simulink model "TrafficLightDecisionLogic"  (R2022b)
settings: Solver=ode23tb  StartTime=0.0  StopTime=scenario.StopTime  FixedStep=0.001  RelTol=1e-8  EnableMultiTasking=on
undefined symbols (not defined in the file or in its folder): maxMIOLeadDistance, posSelector, referencePathSwitchThreshold, Ts, velSelector
settings Model: Creator=The MathWorks, Inc.  LastModifiedBy=The MathWorks, Inc.
settings SolverCC: ZeroCrossAlgorithm=Adaptive  AlgebraicLoopSolver=TrustRegion  PositivePriorityOrder=on  AutoInsertRateTranBlk=on  InsertRTBMode=Always  DecoupledContinuousIntegration=on  MinimalZcImpactIntegration=on  MaxZcPerStep=1
settings DataIOCC: SaveOutput=off  SaveTime=off  ReturnWorkspaceOutputs=off
settings DebuggingCC: ParameterPrecisionLossMsg=none  UnconnectedInputMsg=warning  UnconnectedOutputMsg=warning  UnconnectedLineMsg=warning  PregeneratedLibrarySubsystemCodeDiagnostic=none  SFMachineParentedDataDiag=warning  ArithmeticOperatorsInVariantConditions=warning
settings HardwareCC: ProdLongLongMode=on
settings ModelReferenceCC: EnableRefExpFcnMdlSchedulingChecks=on
settings SFSimCC: SimUseLocalCustomCode=off
settings RTWCC: GenerateReport=on  RTWUseLocalCustomCode=off  LaunchReport=on  DLArmComputeVersion=19.05
settings ConfigComp: CovScope=ReferencedModels  CovIncludeTopModel=off

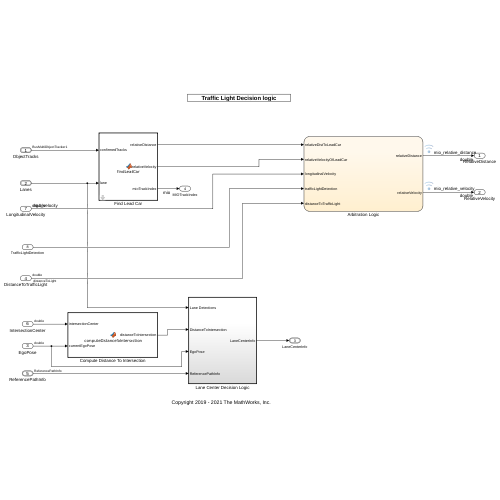
[thumbnail: Simulink's stored preview of the top-level diagram]
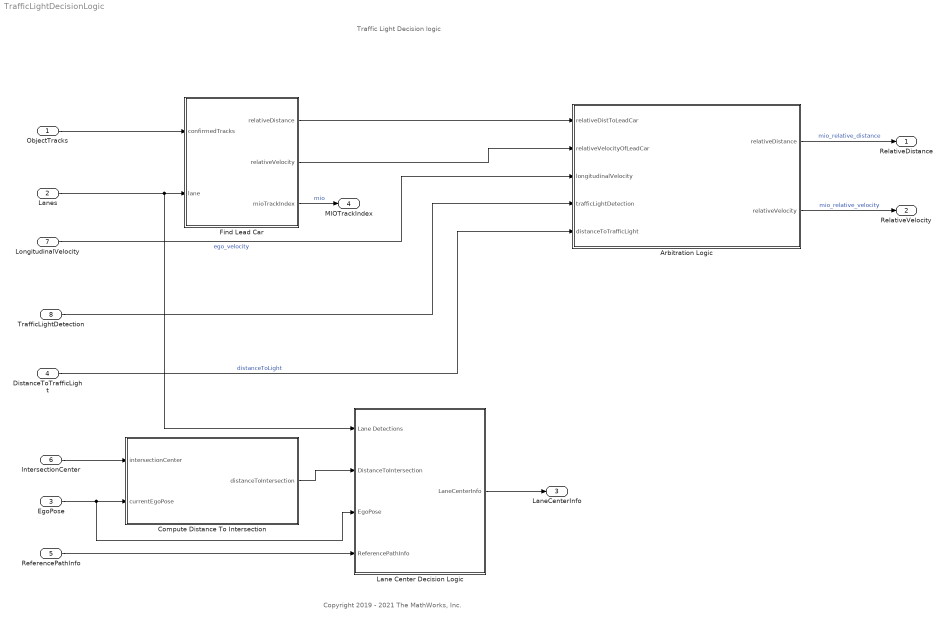
== system TrafficLightDecisionLogic ==
  note: Traffic Light Decision logic
  note: Copyright 2019 - 2021 The MathWorks, Inc.
  ObjectTracks : Inport  OutDataTypeStr=Bus: BusMultiObjectTracker1  PortDimensions=[1 1]  SampleTime=[0.10000000000000001,0]  BusOutputAsStruct=on
  Lanes : Inport  Port=2  OutDataTypeStr=Bus: LaneSensor
  "EgoPose " : Inport  Port=3  OutDataTypeStr=double  PortDimensions=3  SampleTime=[0.10000000000000001,0]
  DistanceToTrafficLight : Inport  Port=4  OutDataTypeStr=double  PortDimensions=1  SampleTime=[0.10000000000000001,0]
  "ReferencePathInfo " : Inport  Port=5  OutDataTypeStr=Bus: ReferencePathInfo  PortDimensions=1  SampleTime=[0.10000000000000001,0]  BusOutputAsStruct=on
  IntersectionCenter : Inport  Port=6  OutDataTypeStr=double  PortDimensions=3  SampleTime=[0.10000000000000001,0]
  LongitudinalVelocity : Inport  Port=7  OutDataTypeStr=double  PortDimensions=1  SampleTime=[0.10000000000000001,0]
  TrafficLightDetection : Inport  Port=8
  Arbitration Logic : Stateflow chart  TreatAsAtomicUnit=on  SystemSampleTime=Ts
  Compute Distance To Intersection : MATLAB Function  TreatAsAtomicUnit=on
  Find Lead Car : MATLAB Function  TreatAsAtomicUnit=on  SystemSampleTime=Ts  mask{positionSelector=posSelector, velocitySelector=velSelector, maxDistance=maxMIOLeadDistance}
      mask prompts: positionSelector "Track position selector"; velocitySelector "Track velocity selector"; maxDistance "Maximum lead distance"
  Lane Center Decision Logic : Subsystem  TreatAsAtomicUnit=on  VariantControl=v2
      settings: RTWFileNameOpts=Use function name
  RelativeDistance : Outport  OutDataTypeStr=double  PortDimensions=1  SampleTime=[0.10000000000000001,0]  VectorParamsAs1DForOutWhenUnconnected=off
  RelativeVelocity : Outport  Port=2  OutDataTypeStr=double  PortDimensions=1  SampleTime=[0.10000000000000001,0]  VectorParamsAs1DForOutWhenUnconnected=off
  LaneCenterInfo : Outport  Port=3  OutDataTypeStr=Bus: BusLaneCenter
  MIOTrackIndex : Outport  Port=4
  wires:
  IntersectionCenter/1 -> Compute Distance To Intersection/1(intersectionCenter)
  LongitudinalVelocity/1 -> Arbitration Logic/3(longitudinalVelocity)  "ego_velocity"
  "ReferencePathInfo "/1 -> Lane Center Decision Logic/4(ReferencePathInfo)
  ObjectTracks/1 -> Find Lead Car/1(confirmedTracks)
  Lanes/1 -> Lane Center Decision Logic/1(Lane Detections), Find Lead Car/2(lane)
  Find Lead Car/3(mioTrackIndex) -> MIOTrackIndex/1  "mio"
  "EgoPose "/1 -> Lane Center Decision Logic/3(EgoPose), Compute Distance To Intersection/2(currentEgoPose)
  Arbitration Logic/1(relativeDistance) -> RelativeDistance/1  "mio_relative_distance"
  Arbitration Logic/2(relativeVelocity) -> RelativeVelocity/1  "mio_relative_velocity"
  Compute Distance To Intersection/1(distanceToIntersection) -> Lane Center Decision Logic/2(DistanceToIntersection)
  Lane Center Decision Logic/1(LaneCenterInfo) -> LaneCenterInfo/1
  TrafficLightDetection/1 -> Arbitration Logic/4(trafficLightDetection)
  Find Lead Car/2(relativeVelocity) -> Arbitration Logic/2(relativeVelocityOfLeadCar)
  DistanceToTrafficLight/1 -> Arbitration Logic/5(distanceToTrafficLight)  "distanceToLight"
  Find Lead Car/1(relativeDistance) -> Arbitration Logic/1(relativeDistToLeadCar)

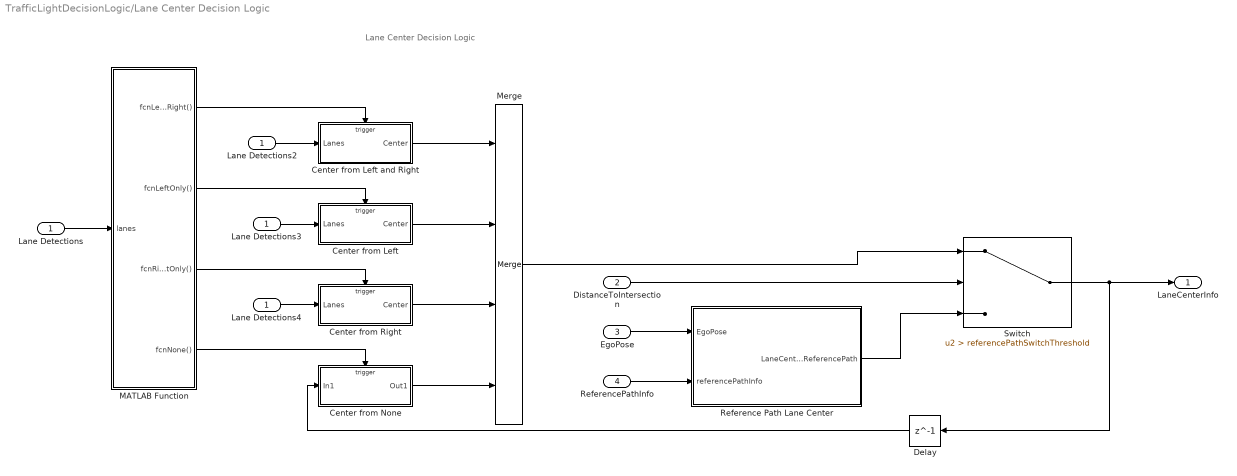
== system TrafficLightDecisionLogic/Lane Center Decision Logic ==
  note: Lane Center Decision Logic
  Lane Detections : Inport
  DistanceToIntersection : Inport  Port=2
  EgoPose : Inport  Port=3
  ReferencePathInfo : Inport  Port=4
  Center from Left : Subsystem  TreatAsAtomicUnit=on
  Center from Left and Right : Subsystem  TreatAsAtomicUnit=on
  Center from None : Subsystem  TreatAsAtomicUnit=on
  Center from Right : Subsystem  TreatAsAtomicUnit=on
  Delay : Delay  DelayLength=1
  Lane Detections2 : InportShadow
  Lane Detections3 : InportShadow
  Lane Detections4 : InportShadow
  MATLAB Function : MATLAB Function  TreatAsAtomicUnit=on
  Merge : Merge  Inputs=4
  Reference Path Lane Center : Subsystem
  Switch : Switch  Criteria=u2 > Threshold  Threshold=referencePathSwitchThreshold  SaturateOnIntegerOverflow=off  InputSameDT=off
      settings: AttributesFormatString=|
      | ----------------------------------------
      | Threshold = %<Threshold>
  LaneCenterInfo : Outport  VectorParamsAs1DForOutWhenUnconnected=off
  wires:
  Center from Right/1(Center) -> Merge/3
  Lane Detections3/1 -> Center from Left/1(Lanes)
  Lane Detections4/1 -> Center from Right/1(Lanes)
  MATLAB Function/2(fcnLeftOnly()) -> Center from Left/Trigger
  MATLAB Function/1(fcnLeftAndRight()) -> Center from Left and Right/Trigger
  Delay/1 -> Center from None/1(In1)
  Center from Left and Right/1(Center) -> Merge/1
  Lane Detections/1 -> MATLAB Function/1(lanes)
  Lane Detections2/1 -> Center from Left and Right/1(Lanes)
  MATLAB Function/3(fcnRightOnly()) -> Center from Right/Trigger
  MATLAB Function/4(fcnNone()) -> Center from None/Trigger
  Center from Left/1(Center) -> Merge/2
  Center from None/1(Out1) -> Merge/4
  ReferencePathInfo/1 -> Reference Path Lane Center/2(referencePathInfo)
  Reference Path Lane Center/1(LaneCenterFromReferencePath) -> Switch/3
  Merge/1 -> Switch/1
  Switch/1 -> LaneCenterInfo/1, Delay/1
  EgoPose/1 -> Reference Path Lane Center/1("EgoPose ")
  DistanceToIntersection/1 -> Switch/2

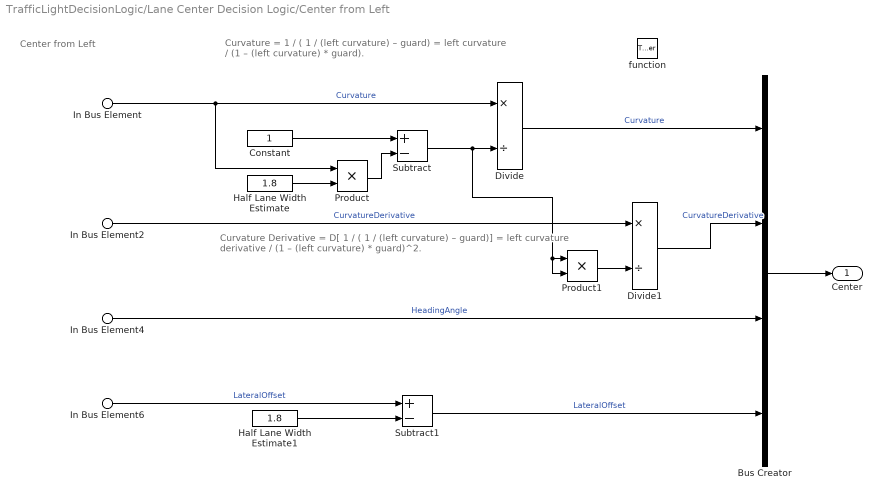
== system TrafficLightDecisionLogic/Lane Center Decision Logic/Center from Left ==
  note: Curvature Derivative
      | = D[ 1 / ( 1 / (left curvature) – guard)]
      | = left curvature derivative / (1 – (left curvature) * guard)^2.
  note: Center from Left
  note: Curvature
      | = 1 / ( 1 / (left curvature) – guard)
      | = left curvature / (1 – (left curvature) * guard).
  In Bus Element : Inport  PortName=Lanes  Element=Left.Curvature
  In Bus Element2 : Inport  PortName=Lanes  Element=Left.CurvatureDerivative
  In Bus Element4 : Inport  PortName=Lanes  Element=Left.HeadingAngle
  In Bus Element6 : Inport  PortName=Lanes  Element=Left.LateralOffset
  function : TriggerPort  TriggerType=function-call  VariantControl=Variant
  Bus Creator : BusCreator  Inputs=4
  Constant : Constant  OutDataTypeStr=Inherit: Inherit via back propagation
  Divide : Product  Inputs=*/
  Divide1 : Product  Inputs=*/
  Half Lane Width Estimate : Constant  Value=1.8  OutDataTypeStr=Inherit: Inherit via back propagation
  Half Lane Width Estimate1 : Constant  Value=1.8  OutDataTypeStr=Inherit: Inherit via back propagation
  Product : Product
  Product1 : Product
  Subtract : Sum  Inputs=+-
  Subtract1 : Sum  Inputs=+-
  Center : Outport  VectorParamsAs1DForOutWhenUnconnected=off
  wires:
  Product/1 -> Subtract/2
  Half Lane Width Estimate1/1 -> Subtract1/2
  In Bus Element6/1 -> Subtract1/1  "LateralOffset"
  Product1/1 -> Divide1/2
  In Bus Element2/1 -> Divide1/1  "CurvatureDerivative"
  Constant/1 -> Subtract/1
  Half Lane Width Estimate/1 -> Product/2
  Subtract/1 -> Divide/2, Product1/1, Product1/2
  In Bus Element/1 -> Divide/1, Product/1  "Curvature"
  Subtract1/1 -> Bus Creator/4  "LateralOffset"
  In Bus Element4/1 -> Bus Creator/3  "HeadingAngle"
  Divide/1 -> Bus Creator/1  "Curvature"
  Divide1/1 -> Bus Creator/2  "CurvatureDerivative"
  Bus Creator/1 -> Center/1

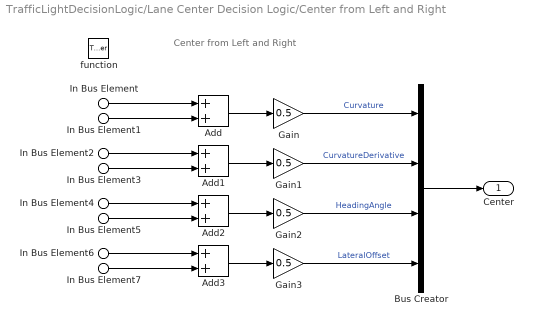
== system TrafficLightDecisionLogic/Lane Center Decision Logic/Center from Left and Right ==
  note: Center from Left and Right
  In Bus Element : Inport  PortName=Lanes  Element=Left.Curvature
  In Bus Element2 : Inport  PortName=Lanes  Element=Left.CurvatureDerivative
  In Bus Element4 : Inport  PortName=Lanes  Element=Left.HeadingAngle
  In Bus Element6 : Inport  PortName=Lanes  Element=Left.LateralOffset
  In Bus Element1 : Inport  PortName=Lanes  Element=Right.Curvature
  In Bus Element3 : Inport  PortName=Lanes  Element=Right.CurvatureDerivative
  In Bus Element5 : Inport  PortName=Lanes  Element=Right.HeadingAngle
  In Bus Element7 : Inport  PortName=Lanes  Element=Right.LateralOffset
  function : TriggerPort  TriggerType=function-call  VariantControl=Variant
  Add{,1..3} (4 alike) : Sum
  Bus Creator : BusCreator  Inputs=4
  Gain{,1..3} (4 alike) : Gain  Gain=0.5
  Center : Outport  VectorParamsAs1DForOutWhenUnconnected=off
  wires:
  In Bus Element6/1 -> Add3/1
  In Bus Element7/1 -> Add3/2
  In Bus Element5/1 -> Add2/2
  In Bus Element4/1 -> Add2/1
  In Bus Element3/1 -> Add1/2
  In Bus Element2/1 -> Add1/1
  In Bus Element1/1 -> Add/2
  In Bus Element/1 -> Add/1
  Bus Creator/1 -> Center/1
  Gain3/1 -> Bus Creator/4  "LateralOffset"
  Add3/1 -> Gain3/1
  Gain2/1 -> Bus Creator/3  "HeadingAngle"
  Add2/1 -> Gain2/1
  Gain1/1 -> Bus Creator/2  "CurvatureDerivative"
  Add1/1 -> Gain1/1
  Gain/1 -> Bus Creator/1  "Curvature"
  Add/1 -> Gain/1

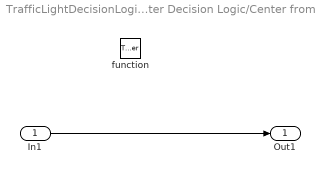
== system TrafficLightDecisionLogic/Lane Center Decision Logic/Center from None ==
  In1 : Inport
  function : TriggerPort  TriggerType=function-call  VariantControl=Variant
  Out1 : Outport  VectorParamsAs1DForOutWhenUnconnected=off
  wires:
  In1/1 -> Out1/1

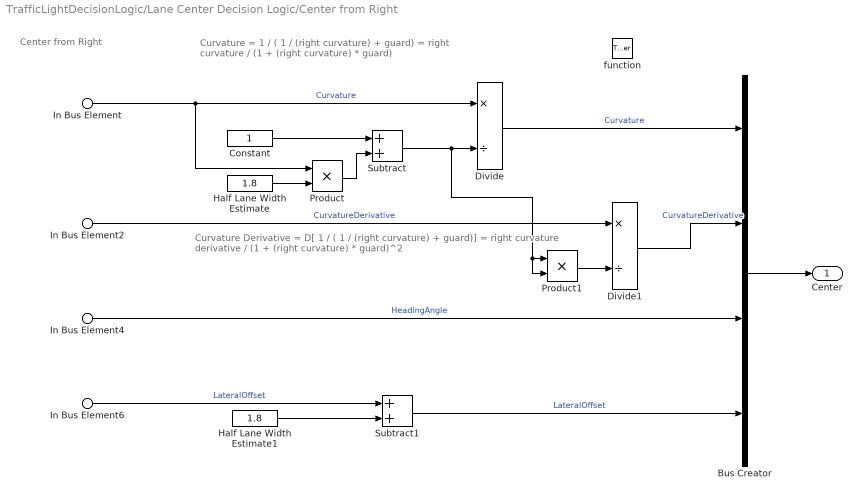
== system TrafficLightDecisionLogic/Lane Center Decision Logic/Center from Right ==
  note: Curvature Derivative
      | = D[ 1 / ( 1 / (right curvature) + guard)]
      | = right curvature derivative / (1 + (right curvature) * guard)^2
  note: Curvature
      | = 1 / ( 1 / (right curvature) + guard)
      | = right curvature / (1 + (right curvature) * guard)
  note: Center from Right
  In Bus Element : Inport  PortName=Lanes  Element=Right.Curvature
  In Bus Element2 : Inport  PortName=Lanes  Element=Right.CurvatureDerivative
  In Bus Element4 : Inport  PortName=Lanes  Element=Right.HeadingAngle
  In Bus Element6 : Inport  PortName=Lanes  Element=Right.LateralOffset
  function : TriggerPort  TriggerType=function-call  VariantControl=Variant
  Bus Creator : BusCreator  Inputs=4
  Constant : Constant  OutDataTypeStr=Inherit: Inherit via back propagation
  Divide : Product  Inputs=*/
  Divide1 : Product  Inputs=*/
  Half Lane Width Estimate : Constant  Value=1.8  OutDataTypeStr=Inherit: Inherit via back propagation
  Half Lane Width Estimate1 : Constant  Value=1.8  OutDataTypeStr=Inherit: Inherit via back propagation
  Product : Product
  Product1 : Product
  Subtract : Sum
  Subtract1 : Sum
  Center : Outport  VectorParamsAs1DForOutWhenUnconnected=off
  wires:
  Half Lane Width Estimate/1 -> Product/2
  Product/1 -> Subtract/2
  Constant/1 -> Subtract/1
  Subtract/1 -> Divide/2, Product1/1, Product1/2
  In Bus Element/1 -> Divide/1, Product/1  "Curvature"
  Bus Creator/1 -> Center/1
  Subtract1/1 -> Bus Creator/4  "LateralOffset"
  Divide/1 -> Bus Creator/1  "Curvature"
  In Bus Element6/1 -> Subtract1/1  "LateralOffset"
  Half Lane Width Estimate1/1 -> Subtract1/2
  In Bus Element4/1 -> Bus Creator/3  "HeadingAngle"
  Product1/1 -> Divide1/2
  Divide1/1 -> Bus Creator/2  "CurvatureDerivative"
  In Bus Element2/1 -> Divide1/1  "CurvatureDerivative"

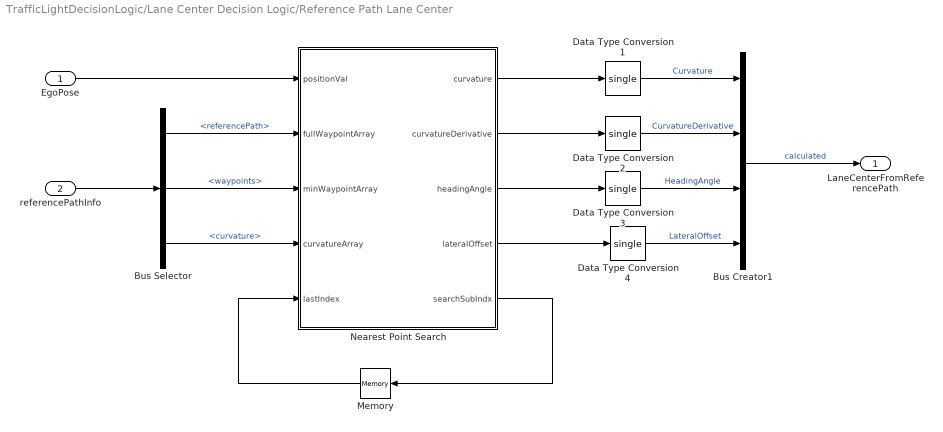
== system TrafficLightDecisionLogic/Lane Center Decision Logic/Reference Path Lane Center ==
  "EgoPose " : Inport
  referencePathInfo : Inport  Port=2
  Bus Creator1 : BusCreator  Inputs=4
  Bus Selector : BusSelector  OutputSignals=referencePath,waypoints,curvature
  Data Type Conversion{1..4} (4 alike) : DataTypeConversion  OutDataTypeStr=single  SaturateOnIntegerOverflow=off  RndMeth=Floor
  Memory : Memory
  Nearest Point Search : MATLAB Function  TreatAsAtomicUnit=on  SystemSampleTime=Ts
  LaneCenterFromReferencePath : Outport
  wires:
  Data Type Conversion4/1 -> Bus Creator1/4  "LateralOffset"
  Bus Selector/3 -> Nearest Point Search/4(curvatureArray)  "<curvature>"
  "EgoPose "/1 -> Nearest Point Search/1(positionVal)
  Data Type Conversion1/1 -> Bus Creator1/1  "Curvature"
  Nearest Point Search/1(curvature) -> Data Type Conversion1/1
  Bus Selector/2 -> Nearest Point Search/3(minWaypointArray)  "<waypoints>"
  Data Type Conversion2/1 -> Bus Creator1/2  "CurvatureDerivative"
  referencePathInfo/1 -> Bus Selector/1
  Nearest Point Search/2(curvatureDerivative) -> Data Type Conversion2/1
  Bus Creator1/1 -> LaneCenterFromReferencePath/1  "calculated"
  Data Type Conversion3/1 -> Bus Creator1/3  "HeadingAngle"
  Nearest Point Search/5(searchSubIndx) -> Memory/1
  Nearest Point Search/3(headingAngle) -> Data Type Conversion3/1
  Nearest Point Search/4(lateralOffset) -> Data Type Conversion4/1
  Bus Selector/1 -> Nearest Point Search/2(fullWaypointArray)  "<referencePath>"
  Memory/1 -> Nearest Point Search/5(lastIndex)

== stateflow chart TrafficLightDecisionLogic/Arbitration Logic ==
  state OnEntry
    entry:
    relativeDistance = relativeDistToLeadCar;
    relativeVelocity = relativeVelocityOfLeadCar;
  state OnRedAndYellowLightDetection
    entry:
    relativeDistance = min(relativeDistToLeadCar,distanceToTrafficLight);
    relativeVelocity = min(relativeVelocityOfLeadCar,longitudinalVelocity);
  (default) -> OnEntry
  OnEntry -> OnEntry [order 2] : [hasChanged(relativeDistToLeadCar)]
  OnRedAndYellowLightDetection -> OnEntry [order 1] : [trafficLightDetection==Green || trafficLightDetection == NoDetections  ]
  OnEntry -> OnRedAndYellowLightDetection [order 1] : [(trafficLightDetection==Red || trafficLightDetection==Yellow) && distanceToTrafficLight ~= inf]
  OnRedAndYellowLightDetection -> OnRedAndYellowLightDetection [order 2] : [hasChanged(relativeDistToLeadCar)]
  OnRedAndYellowLightDetection -> OnRedAndYellowLightDetection [order 3] : [hasChanged(distanceToTrafficLight)]
  data: relativeDistance output; relativeDistToLeadCar input; relativeVelocityOfLeadCar input; longitudinalVelocity input; trafficLightDetection input; distanceToTrafficLight input; relativeVelocity output; Green local =2; Red local =0; Yellow local =1; NoDetections local =-1

== matlab function TrafficLightDecisionLogic/Lane Center Decision Logic/MATLAB Function ==
  data: lanes input
  events: fcnLeftAndRight output FUNCTION_CALL_EVENT; fcnLeftOnly output FUNCTION_CALL_EVENT; fcnRightOnly output FUNCTION_CALL_EVENT; fcnNone output FUNCTION_CALL_EVENT
function fcn(lanes)

leftStrength  = lanes.Left.Strength;
rightStrength = lanes.Right.Strength;

if (leftStrength > 0) && (rightStrength > 0)
   fcnLeftAndRight();
   
elseif leftStrength > 0
    fcnLeftOnly();
    
elseif rightStrength > 0
    fcnRightOnly();
    
else
    fcnNone();
end

== matlab function TrafficLightDecisionLogic/Lane Center Decision Logic/Reference Path Lane Center/Nearest Point Search ==
  data: curvature output; positionVal input; fullWaypointArray input; minWaypointArray input; curvatureDerivative output; headingAngle output; lateralOffset output; curvatureArray input; searchSubIndx output; lastIndex input
function [curvature, curvatureDerivative, headingAngle, lateralOffset, searchSubIndx] = nearestPointSearch(positionVal, fullWaypointArray, minWaypointArray,  curvatureArray, lastIndex)
% curvature = initial curvature per unit length                  [1/m]
% curvatureDerivative = (constant) derivative of curvature per unit length [1/m^2]
% headingAngle = Relative heading angle of vehicle wrt Lane [rad]
% lateralOffset  = offset of vehicle from center of the lane [m]
% searchSubIndx = Index of last search

minArraySize = max(size(minWaypointArray));
fullArraySize = max(size(fullWaypointArray));

% Initialize dmin with a uint32 maximum value.
dmin = double(intmax('uint32'));

% Default interpolation points for clothoid fitting.
interpolationPoints = 1024;

% Get current location
yawVal = positionVal(3)*pi/180;
searchIndx = floor(lastIndex / interpolationPoints);
if(searchIndx < 1 )
    searchIndx = 1;
end
nearestDataPoint = [0 0];

% Look for the closest point in the smaller waypoints set
for indx = searchIndx:minArraySize
    
    % find the closest point in the bigger matrix.
    point1 = [minWaypointArray(indx,1) minWaypointArray(indx,2)];
    
    % checking eucledian distance of point from the line.
    distance = sqrt((point1(1)-positionVal(1))^2 + (point1(2) - positionVal(2))^2 );
    if (distance <= dmin)
        searchIndx = double(indx);
        dmin = distance;
        nearestDataPoint = point1;
    end
end
sectionIndex = searchIndx;

% Increment the index by one so as not to have invalid equations.
searchSubIndx = lastIndex + 1 ;

% Search in the near by location of the search index.
lowerSearchLimit = (sectionIndex-1) * interpolationPoints;
if((sectionIndex-1) < 1)
    lowerSearchLimit  = 1;
end
upperSearchLimit = fullArraySize;
if((sectionIndex + 2) * interpolationPoints < fullArraySize)
    upperSearchLimit  = (sectionIndex + 2) * interpolationPoints;
end

% search loop
for indx = lowerSearchLimit:5:upperSearchLimit
    if(indx < fullArraySize)
        % get the point in the full waypoints array
        point1 = [fullWaypointArray(indx,1) fullWaypointArray(indx,2)];
        % checking eucledian distance of point from the line.
        distance = sqrt((point1(1) - positionVal(1))^2 + (point1(2)-positionVal(2))^2 );
        if (distance <= dmin)
            searchSubIndx = double(indx);
            dmin = distance;
            nearestDataPoint = point1;
        end
    else
        % get the point in the waypoints array
        point1 = [fullWaypointArray(indx,1) fullWaypointArray(indx,2)];
        % checking eucledian distance of point from the line.
        distance = sqrt((point1(1)-positionVal(1))^2 + (point1(2)-positionVal(2))^2 );
        if (distance <= dmin)
            searchSubIndx = double(indx);
            dmin = distance;
            nearestDataPoint = point1;
        end
    end
end

% To obtain relative heading Angle, we need to subtract the current yaw
% angle of the vehicle from the current angle of the lane. This gives us
% our relative yaw angle.
% We need to compute the directionality of the our doffset. This can be
% done easily by checking on which side of a straight line formed by lane
% points does the current postion is.
% First, find the slope of the line.
if(searchSubIndx >= fullArraySize)
    searchSubIndx = fullArraySize;
end
% Increase the index by 5 to make it not to look in the same index.
nextIndx = searchSubIndx + 5;
if(nextIndx >= fullArraySize)
    nextIndx = fullArraySize;
end

% find the projection of position on the line joining the two waypoints
% this results in more accurate calcualtion of lateralOffset.
point1 = [nearestDataPoint(1) nearestDataPoint(2)];
point2 = [fullWaypointArray(nextIndx, 1) fullWaypointArray(nextIndx, 2)];
diffPoint = point2 - point1;

% obtain the slope of line connecting the two waypoints, this is also the
% lane angle.
laneAngleValue = atan2(diffPoint(2) , diffPoint(1));

% Finding the perpendicular distance to the line connecting two waypoints
% and the point given using the given formula
% Line: Ax + By + C = 0;
% Pt: P = (x1, y1)
% Dist: |Ax1 + By1 + C| / (A^2 + B^2)^1/2
%
% Here the line is of the format: mx - y + c =0
% this results in two special cases when m = 0 or inf
m1 = tan(laneAngleValue);
if(abs(m1) <= 1e-02)
    c1 = point1(2);
    doffset = abs(- positionVal(2) + c1);
elseif(m1 == inf || m1 == -inf )
    c1 = - point1(1);
    doffset = abs(positionVal(1) + c1);
else
    c1 = point1(2) - m1 * point1(1);
    doffset = abs(m1 * positionVal(1) - positionVal(2) + c1)...
        / sqrt(1 + m1 * m1);
end

% Finding the direction of the point with respect to the line. This is
% using the vector algebra, by the sign of the cross product bwtween two
% vectors.
% AB X AP > 0 for anticlockwise angle b/w AB and AP
% AB X AP < 0 for clockwise angle b/w AB and AP
% The line is formed by pts
%   A = (x1,y1)
%   B = (x2,y2)
% We are testing for point P = (x,y)
%  sign = (x−x1)(y2−y1)−(y−y1)(x2−x1) > 0  for RHS; (anticlockwise motion)
%  sign = (x−x1)(y2−y1)−(y−y1)(x2−x1) < 0  for LHS; (clockwise motion)
sign = (positionVal(1) - point1(1)) * (point2(2) - point1(2)) ...
    - (positionVal(2) -  point1(2)) * (point2(1) - point1(1));

% set the direction of doffset if the point is on LHS( -ve doffset)
if(sign < 0)
    doffset = -1 * doffset;
end

curvature =  curvatureArray(searchSubIndx);
if(searchSubIndx ~= fullArraySize)
    curvatureDerivative = curvatureArray(searchSubIndx + 1) - curvatureArray(searchSubIndx);
else
    curvatureDerivative = curvatureArray(end) - curvatureArray(end - 1);
end

% assign the value to the output variables
lateralOffset = doffset;
headingAngle = laneAngleValue - yawVal;

% Wrap up Heading Angle to (-pi, pi)
if ( headingAngle > pi)
    headingAngle = - 2 * pi + headingAngle ;
elseif( headingAngle < - pi)
    headingAngle = 2 * pi + headingAngle;
end
end

== matlab function TrafficLightDecisionLogic/Compute Distance To Intersection ==
  data: intersectionCenter input; distanceToIntersection output; currentEgoPose input
function distanceToIntersection = computeDistanceToIntersection(intersectionCenter, currentEgoPose)

distanceToIntersection = double(sqrt((intersectionCenter(1)- ...
    currentEgoPose(1))^2 + (intersectionCenter(2)- currentEgoPose(2))^2));

end

== matlab function TrafficLightDecisionLogic/Find Lead Car ==
  data: confirmedTracks input; relativeDistance output size=[1 1]; relativeVelocity output size=[1 1]; lane input; mioTrackIndex output; positionSelector parameter; maxDistance parameter; velocitySelector parameter
function [relativeDistance,relativeVelocity,mioTrackIndex] = findLeadCar(confirmedTracks, lane, positionSelector, maxDistance, velocitySelector)
% This function finds the lead car: a car in front of the ego car that
% satisfies all the criteria below:
% * Within the ego car's lane.
% * In front of the ego car.
% * Closest to the ego car.

% Note: If you change state definition, change the following:
%       State = [x;vx;y;vy;z;vz] (3D constant velocity)

% Copyright 2019-2021 The MathWorks, Inc.

[relativeDistance,relativeVelocity,mioTrackIndex] = helperFindMIOTrack(confirmedTracks, lane, positionSelector, velocitySelector, maxDistance);
